simulink model "MultirotorSimPx4"  (R2018b)
settings: Solver=VariableStepAuto  StartTime=0.0  StopTime=Simulation.T_END  MaxStep=Simulation.TS_MAX  RelTol=1e-3  EnableMultiTasking=on
PreLoadFcn:
  | % InitializeParameters;
undefined symbols (not defined in the file): Aero, Initial, Motor, Simulation, Uav
libraries: QuaternionLibrary x13, simulink_extras x9, Px4Library x4, simulink x1
(part 5 of 8)

== matlab function MultirotorSimPx4/Sensor Model/local_position_estimator/Input assignment ==
  data: armed_armed input; att_q input; mocap_timestamp input; mocap_updated input; mocap_x input; mocap_y input; mocap_z input; sensor_accelerometer_m_s2 input; sensor_baro_alt_meter input; sensor_baro_timestamp_relative input; sensor_timestamp input; sensor_updated input; selfVecIn input; selfVec output
function selfVec = InputAssignment( ...
	                             armed_armed, ...
	                                   att_q, ...
	                         mocap_timestamp, ...
	                           mocap_updated, ...
	                                 mocap_x, ...
	                                 mocap_y, ...
	                                 mocap_z, ...
	               sensor_accelerometer_m_s2, ...
	                   sensor_baro_alt_meter, ...
	          sensor_baro_timestamp_relative, ...
	                        sensor_timestamp, ...
	                          sensor_updated, ...
	                               selfVecIn ...
	)
%#codegen

	selfVec = selfVecIn;

	% Variable assignment
	selfVec(518:518) =                              armed_armed;
	selfVec(519:522) =                                    att_q;
	selfVec(530:530) =                          mocap_timestamp;
	selfVec(531:531) =                            mocap_updated;
	selfVec(532:532) =                                  mocap_x;
	selfVec(533:533) =                                  mocap_y;
	selfVec(534:534) =                                  mocap_z;
	selfVec(537:539) =                sensor_accelerometer_m_s2;
	selfVec(540:540) =                    sensor_baro_alt_meter;
	selfVec(541:541) =           sensor_baro_timestamp_relative;
	selfVec(542:542) =                         sensor_timestamp;
	selfVec(543:543) =                           sensor_updated;
end

== matlab function MultirotorSimPx4/Sensor Model/local_position_estimator/Output selection ==
  data: est_status_covariances output; est_status_health_flags output; est_status_states output; gpos_vel_n output; gpos_vel_e output; selfVec input; gpos_vel_d output; lpos_vx output; lpos_vy output; lpos_vz output; lpos_x output; lpos_y output; lpos_z output; lpos_yaw output
function [ ...
                   est_status_covariances, ...
                  est_status_health_flags, ...
                        est_status_states, ...
                               gpos_vel_n, ...
                               gpos_vel_e, ...
                               gpos_vel_d, ...
                                  lpos_vx, ...
                                  lpos_vy, ...
                                  lpos_vz, ...
                                   lpos_x, ...
                                   lpos_y, ...
                                   lpos_z, ...
                                 lpos_yaw] ...
   = OutputSelection( selfVec )
%#codegen

	% Variable assignment
	                  est_status_covariances = selfVec(439:448);
	                 est_status_health_flags = selfVec(449:449);
	                       est_status_states = selfVec(454:463);
	                              gpos_vel_n = selfVec(480:480);
	                              gpos_vel_e = selfVec(481:481);
	                              gpos_vel_d = selfVec(482:482);
	                                 lpos_vx = selfVec(501:501);
	                                 lpos_vy = selfVec(502:502);
	                                 lpos_vz = selfVec(503:503);
	                                  lpos_x = selfVec(504:504);
	                                  lpos_y = selfVec(507:507);
	                                  lpos_z = selfVec(508:508);
	                                lpos_yaw = selfVec(512:512);
end
